simulink model "joint_trajectory_planner"  (R2020a)
settings: Solver=ode3  StartTime=0.0  StopTime=inf  FixedStep=0.01  RelTol=1e-3
libraries: robotlib x20, robotcorelib x1
settings Model: Creator=paolo  LastModifiedBy=paolo
settings OptimizationCC: EnhancedBackFolding=on  PassReuseOutputArgsAs=Individual arguments  ZeroExternalMemoryAtStartup=off  ZeroInternalMemoryAtStartup=off  MaxStackSize=64  OptimizeBlockOrder=speed  DifferentSizesBufferReuse=on  OptimizationCustomize=off  EfficientTunableParamExpr=on
settings DebuggingCC: ParameterTunabilityLossMsg=error
settings HardwareCC: ProdBitPerPointer=32  ProdBitPerSizeT=32  ProdBitPerPtrDiffT=32  ProdLargestAtomicFloat=None  ProdIntDivRoundTo=Undefined  ProdEndianess=Unspecified  ProdWordSize=32  ProdHWDeviceType=Generic->Unspecified (assume 32-bit Generic)
settings SFSimCC: MATLABDynamicMemAlloc=off
settings RTWCC: SystemTargetFile=ert.tlc  HardwareBoard=Robot Operating System (ROS)  TemplateMakefile=ert_default_tmf  Toolchain=Catkin  TargetLang=C++
settings CodeAppCC: ForceParamTrailComments=on  IgnoreCustomStorageClasses=off  OperatorAnnotations=on  SimulinkDataObjDesc=on  SFDataObjDesc=on  InsertBlockDesc=on

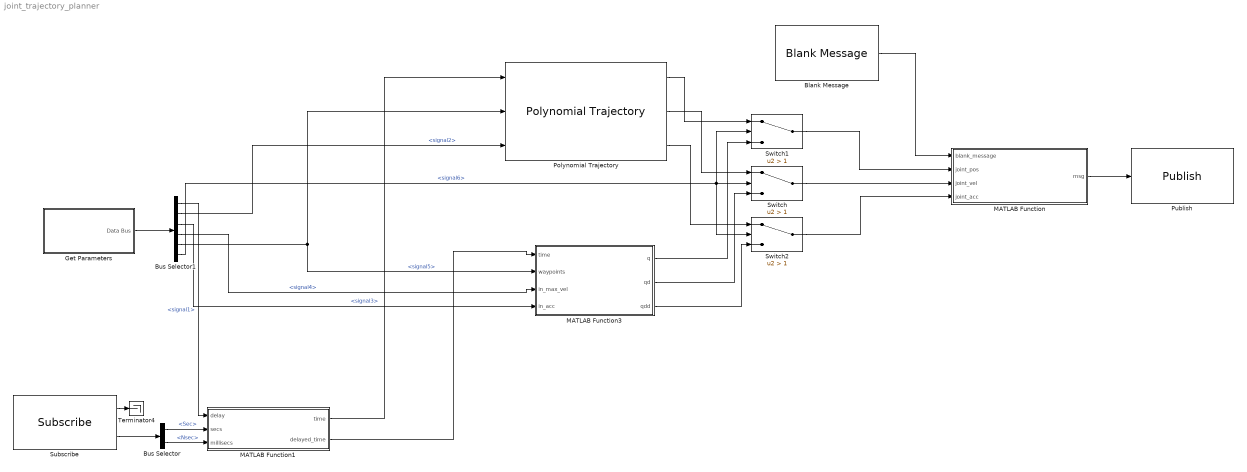
== system joint_trajectory_planner ==
  Blank Message : robotlib/Blank Message  messageClass=Message  entityType=trajectory_msgs/JointTrajectoryPoint  messageType=trajectory_msgs/JointTrajectoryPoint  SampleTime=-1
  Bus Selector : BusSelector  OutputSignals=Clock_.Sec,Clock_.Nsec
  Bus Selector1 : BusSelector  OutputSignals=signal1,signal2,signal3,signal4,signal5,signal6
  Get Parameters : Subsystem
  MATLAB Function : MATLAB Function  TreatAsAtomicUnit=on
  MATLAB Function1 : MATLAB Function  TreatAsAtomicUnit=on
  MATLAB Function3 : MATLAB Function  TreatAsAtomicUnit=on
  Polynomial Trajectory : robotcorelib/Polynomial Trajectory  WaypointSource=External  Waypoints=[ 0, 2, 1, 5, 0; -1, 3, 1, 4, 4 ]  TimePoints=[ 0, 1, 2, 3, 4 ]  TimeInterval=[ 1, 4 ]  Method=Cubic Polynomial  ParameterSource=Internal  VelocityBoundaryCondition=zeros( 6, 2 )  AccelerationBoundaryCondition=zeros( 2, 5 )  SimulateUsing=Interpreted execution
      settings: SourceProductBaseCode=NV,RO,RR
  Publish : robotlib/Publish  topicSource=Select from ROS network  topic=/joint_trajectory  messageType=trajectory_msgs/JointTrajectoryPoint  messageQueueLength=1
      link override SinkBlock: ROSTopic=/joint_trajectory  ROSMessageType=trajectory_msgs/JointTrajectoryPoint  SLBusName=SL_Bus_joint_trajectory_planner_JointTrajectoryPoint_y0wep  ModelName=joint_trajectory_planner  BlockId=Pub_joint_trajectory_planner_5
  Subscribe : robotlib/Subscribe  topicSource=Specify your own  topic=/clock  messageType=rosgraph_msgs/Clock  sampleTime=-1  messageQueueLength=1
  Switch : Switch  Criteria=u2 > Threshold  Threshold=1
  Switch1 : Switch  Criteria=u2 > Threshold  Threshold=1
  Switch2 : Switch  Criteria=u2 > Threshold  Threshold=1
  Terminator4 : Terminator
  wires:
  MATLAB Function/1(msg) -> Publish/1
  MATLAB Function3/2(qd) -> Switch/3
  Subscribe/1 -> Terminator4/1
  Subscribe/2 -> Bus Selector/1
  Bus Selector/1 -> MATLAB Function1/2(secs)  "<Sec>"
  Bus Selector/2 -> MATLAB Function1/3(millisecs)  "<Nsec>"
  MATLAB Function1/1(time) -> Polynomial Trajectory/1
  MATLAB Function3/1(q) -> Switch1/3
  MATLAB Function3/3(qdd) -> Switch2/3
  Get Parameters/1(Data Bus) -> Bus Selector1/1
  Bus Selector1/1 -> MATLAB Function1/1(delay)  "<signal1>"
  Bus Selector1/2 -> Polynomial Trajectory/3  "<signal2>"
  Bus Selector1/5 -> MATLAB Function3/2(waypoints), Polynomial Trajectory/2  "<signal5>"
  Blank Message/1 -> MATLAB Function/1(blank_message)
  Switch1/1 -> MATLAB Function/2(joint_pos)
  Switch/1 -> MATLAB Function/3(joint_vel)
  Switch2/1 -> MATLAB Function/4(joint_acc)
  Polynomial Trajectory/2 -> Switch/1
  Polynomial Trajectory/3 -> Switch2/1
  Bus Selector1/6 -> Switch2/2, Switch1/2, Switch/2  "<signal6>"
  MATLAB Function1/2(delayed_time) -> MATLAB Function3/1(time)
  Bus Selector1/4 -> MATLAB Function3/3(in_max_vel)  "<signal4>"
  Polynomial Trajectory/1 -> Switch1/1
  Bus Selector1/3 -> MATLAB Function3/4(in_acc)  "<signal3>"

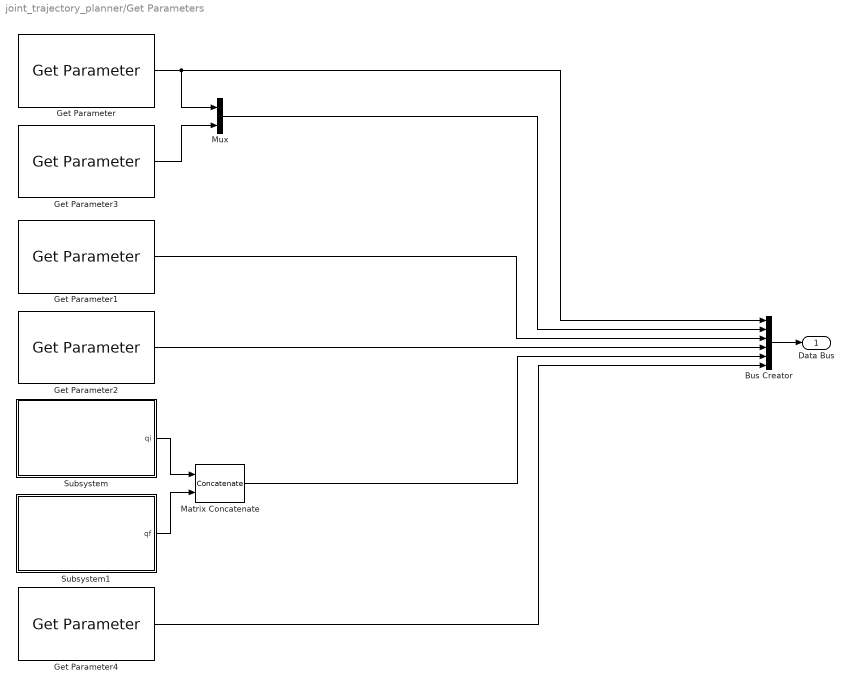
== system joint_trajectory_planner/Get Parameters ==
  Bus Creator : BusCreator  Inputs=6
  Get Parameter : robotlib/Get Parameter  ParameterSource=Specify your own  ParameterName=/start_delay  ParameterType=double  ParameterMaxArrayLength=16  ParameterInitialValue=20  SampleTime=-1  ShowErrorCodeOutput=off  ModelName=joint_trajectory_planner  BlockId=ParamGet_joint_trajectory_planner_26
      settings: SourceProductBaseCode=RR
  Get Parameter1 : robotlib/Get Parameter  ParameterSource=Specify your own  ParameterName=/max_ang_acc  ParameterType=double  ParameterMaxArrayLength=16  ParameterInitialValue=1  SampleTime=-1  ShowErrorCodeOutput=off  ModelName=joint_trajectory_planner  BlockId=ParamGet_joint_trajectory_planner_27
      settings: SourceProductBaseCode=RR
  Get Parameter2 : robotlib/Get Parameter  ParameterSource=Specify your own  ParameterName=/max_ang_vel  ParameterType=double  ParameterMaxArrayLength=16  ParameterInitialValue=1  SampleTime=-1  ShowErrorCodeOutput=off  ModelName=joint_trajectory_planner  BlockId=ParamGet_joint_trajectory_planner_28
      settings: SourceProductBaseCode=RR
  Get Parameter3 : robotlib/Get Parameter  ParameterSource=Specify your own  ParameterName=/tf  ParameterType=double  ParameterMaxArrayLength=16  ParameterInitialValue=60  SampleTime=-1  ShowErrorCodeOutput=off  ModelName=joint_trajectory_planner  BlockId=ParamGet_joint_trajectory_planner_49
      settings: SourceProductBaseCode=RR
  Get Parameter4 : robotlib/Get Parameter  ParameterSource=Specify your own  ParameterName=/trajectoryType  ParameterType=int32  ParameterMaxArrayLength=16  ParameterInitialValue=1  SampleTime=-1  ShowErrorCodeOutput=off  ModelName=joint_trajectory_planner  BlockId=ParamGet_joint_trajectory_planner_50
      settings: SourceProductBaseCode=RR
  Matrix Concatenate : Concatenate  Mode=Multidimensional array  ConcatenateDimension=2
  Mux : Mux  Inputs=2
  Subsystem : Subsystem
  Subsystem1 : Subsystem
  Data Bus : Outport
  wires:
  Subsystem/1(qi) -> Matrix Concatenate/1
  Subsystem1/1(qf) -> Matrix Concatenate/2
  Get Parameter/1 -> Bus Creator/1, Mux/1
  Get Parameter3/1 -> Mux/2
  Bus Creator/1 -> Data Bus/1
  Mux/1 -> Bus Creator/2
  Get Parameter1/1 -> Bus Creator/3
  Matrix Concatenate/1 -> Bus Creator/5
  Get Parameter4/1 -> Bus Creator/6
  Get Parameter2/1 -> Bus Creator/4

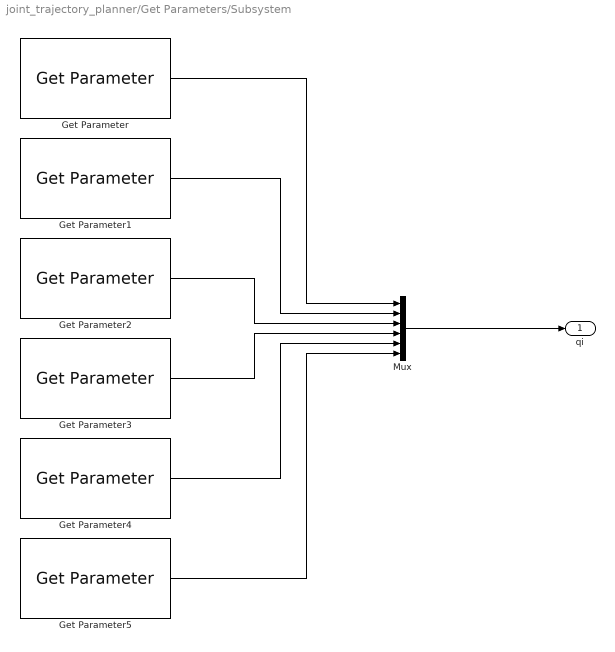
== system joint_trajectory_planner/Get Parameters/Subsystem ==
  Get Parameter : robotlib/Get Parameter  ParameterSource=Specify your own  ParameterName=/q1_initial  ParameterType=double  ParameterMaxArrayLength=16  ParameterInitialValue=0.0  SampleTime=-1  ShowErrorCodeOutput=off  ModelName=joint_trajectory_planner  BlockId=ParamGet_joint_trajectory_planner_34
      settings: SourceProductBaseCode=RR
  Get Parameter1 : robotlib/Get Parameter  ParameterSource=Specify your own  ParameterName=/q2_initial  ParameterType=double  ParameterMaxArrayLength=16  ParameterInitialValue=0.0  SampleTime=-1  ShowErrorCodeOutput=off  ModelName=joint_trajectory_planner  BlockId=ParamGet_joint_trajectory_planner_35
      settings: SourceProductBaseCode=RR
  Get Parameter2 : robotlib/Get Parameter  ParameterSource=Specify your own  ParameterName=/q3_initial  ParameterType=double  ParameterMaxArrayLength=16  ParameterInitialValue=0.0  SampleTime=-1  ShowErrorCodeOutput=off  ModelName=joint_trajectory_planner  BlockId=ParamGet_joint_trajectory_planner_36
      settings: SourceProductBaseCode=RR
  Get Parameter3 : robotlib/Get Parameter  ParameterSource=Specify your own  ParameterName=/q4_initial  ParameterType=double  ParameterMaxArrayLength=16  ParameterInitialValue=0.0  SampleTime=-1  ShowErrorCodeOutput=off  ModelName=joint_trajectory_planner  BlockId=ParamGet_joint_trajectory_planner_37
      settings: SourceProductBaseCode=RR
  Get Parameter4 : robotlib/Get Parameter  ParameterSource=Specify your own  ParameterName=/q5_initial  ParameterType=double  ParameterMaxArrayLength=16  ParameterInitialValue=0.0  SampleTime=-1  ShowErrorCodeOutput=off  ModelName=joint_trajectory_planner  BlockId=ParamGet_joint_trajectory_planner_38
      settings: SourceProductBaseCode=RR
  Get Parameter5 : robotlib/Get Parameter  ParameterSource=Specify your own  ParameterName=/q6_initial  ParameterType=double  ParameterMaxArrayLength=16  ParameterInitialValue=0.0  SampleTime=-1  ShowErrorCodeOutput=off  ModelName=joint_trajectory_planner  BlockId=ParamGet_joint_trajectory_planner_39
      settings: SourceProductBaseCode=RR
  Mux : Mux  Inputs=6
  qi : Outport
  wires:
  Get Parameter/1 -> Mux/1
  Get Parameter1/1 -> Mux/2
  Get Parameter2/1 -> Mux/3
  Get Parameter3/1 -> Mux/4
  Get Parameter4/1 -> Mux/5
  Get Parameter5/1 -> Mux/6
  Mux/1 -> qi/1

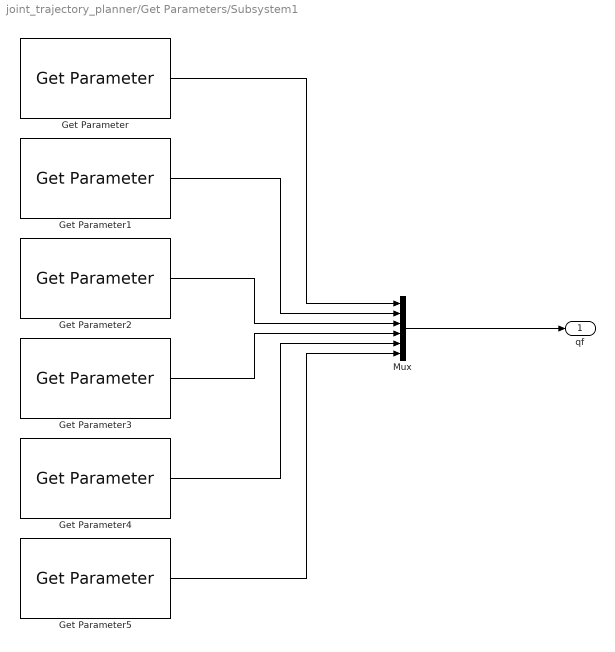
== system joint_trajectory_planner/Get Parameters/Subsystem1 ==
  Get Parameter : robotlib/Get Parameter  ParameterSource=Specify your own  ParameterName=/q1_final  ParameterType=double  ParameterMaxArrayLength=16  ParameterInitialValue=6.28  SampleTime=-1  ShowErrorCodeOutput=off  ModelName=joint_trajectory_planner  BlockId=ParamGet_joint_trajectory_planner_41
      settings: SourceProductBaseCode=RR
  Get Parameter1 : robotlib/Get Parameter  ParameterSource=Specify your own  ParameterName=/q2_final  ParameterType=double  ParameterMaxArrayLength=16  ParameterInitialValue=6.28  SampleTime=-1  ShowErrorCodeOutput=off  ModelName=joint_trajectory_planner  BlockId=ParamGet_joint_trajectory_planner_42
      settings: SourceProductBaseCode=RR
  Get Parameter2 : robotlib/Get Parameter  ParameterSource=Specify your own  ParameterName=/q3_final  ParameterType=double  ParameterMaxArrayLength=16  ParameterInitialValue=6.28  SampleTime=-1  ShowErrorCodeOutput=off  ModelName=joint_trajectory_planner  BlockId=ParamGet_joint_trajectory_planner_43
      settings: SourceProductBaseCode=RR
  Get Parameter3 : robotlib/Get Parameter  ParameterSource=Specify your own  ParameterName=/q4_final  ParameterType=double  ParameterMaxArrayLength=16  ParameterInitialValue=6.28  SampleTime=-1  ShowErrorCodeOutput=off  ModelName=joint_trajectory_planner  BlockId=ParamGet_joint_trajectory_planner_44
      settings: SourceProductBaseCode=RR
  Get Parameter4 : robotlib/Get Parameter  ParameterSource=Specify your own  ParameterName=/q5_final  ParameterType=double  ParameterMaxArrayLength=16  ParameterInitialValue=6.28  SampleTime=-1  ShowErrorCodeOutput=off  ModelName=joint_trajectory_planner  BlockId=ParamGet_joint_trajectory_planner_45
      settings: SourceProductBaseCode=RR
  Get Parameter5 : robotlib/Get Parameter  ParameterSource=Specify your own  ParameterName=/q6_final  ParameterType=double  ParameterMaxArrayLength=16  ParameterInitialValue=6.28  SampleTime=-1  ShowErrorCodeOutput=off  ModelName=joint_trajectory_planner  BlockId=ParamGet_joint_trajectory_planner_46
      settings: SourceProductBaseCode=RR
  Mux : Mux  Inputs=6
  qf : Outport
  wires:
  Get Parameter/1 -> Mux/1
  Get Parameter1/1 -> Mux/2
  Get Parameter2/1 -> Mux/3
  Get Parameter3/1 -> Mux/4
  Get Parameter4/1 -> Mux/5
  Get Parameter5/1 -> Mux/6
  Mux/1 -> qf/1

== matlab function joint_trajectory_planner/MATLAB Function1 ==
  data: delay input; secs input; time output; millisecs input; delayed_time output
function [time, delayed_time] = get_time(delay, secs, millisecs)

    time = secs + millisecs / 1e9;
    delayed_time = time - delay;
    
    if delayed_time < 0
        delayed_time = 0;
    end

== matlab function joint_trajectory_planner/MATLAB Function ==
  data: blank_message input; joint_pos input; msg output Bus: SL_Bus_joint_trajectory_planner_JointTrajectoryPoint_y0wep; joint_vel input; joint_acc input
function msg = assign_trajectory(blank_message, joint_pos, joint_vel, joint_acc)

    msg = blank_message;
    numJoints = length(joint_vel);
    msg.Velocities_SL_Info.CurrentLength = uint32(numJoints);
    msg.Velocities(1:numJoints) = joint_vel;
    msg.Positions_SL_Info.CurrentLength = uint32(numJoints);
    msg.Positions(1:numJoints) = joint_pos;
    msg.Accelerations_SL_Info.CurrentLength = uint32(numJoints);
    msg.Accelerations(1:numJoints) = joint_acc;

== matlab function joint_trajectory_planner/MATLAB Function3 ==
  data: time input; q output; waypoints input; in_max_vel input; in_acc input; qd output; qdd output
function [q, qd, qdd] = fcn(time, waypoints, in_max_vel, in_acc)

q_len = length(waypoints);

q = waypoints(:, 1);
qd = zeros(q_len, 1);
qdd = zeros(q_len, 1);

[rows, columns] = size(waypoints);

if length(in_max_vel) == 1
    max_vel = in_max_vel * ones(q_len, 1);
else
    max_vel = in_max_vel;
end

if length(in_acc) == 1
    acc = in_acc * ones(q_len, 1);
else
    acc = in_acc;
end

act_max_vel = zeros(rows, columns-1);
signes = zeros(rows, columns-1);
t = zeros(rows, columns-1, 3);

for i=1:rows
    
    t_up = max_vel(i) / acc(i);
   
    for j=1:columns-1
        
        dist = waypoints(i, j+1) - waypoints(i, j);
        signes(i, j) = sign(dist);
        
        if abs(dist) < t_up * max_vel(i)
            act_t_up = sqrt(abs(dist)/acc(i));
            t(i, j, 2) = 0;
            t(i, j, 1) = act_t_up;
            t(i, j, 3) = act_t_up;
            act_max_vel(i, j) = act_t_up * acc(i);
        else
            t(i, j, 1) = t_up;
            t(i, j, 3) = t_up;
            t(i, j, 2) = (abs(dist) - t_up * max_vel(i)) / max_vel(i);
            act_max_vel(i, j) = max_vel(i);
        end
        
    end
         
end

for i=1:rows
    
    t1 = time;
    
    for j=1:columns-1
        
        for k=1:3
            
            if t1 - t(i, j, k) < 0
                if k == 1
                    q(i) = q(i) + 1/2* acc(i) * t1^2 * signes(i, j);
                    qd(i) = acc(i) * t1 * signes(i, j);
                    qdd(i) = acc(i) * signes(i, j);
                    t1 = t1 - t(i, j, k);
                    break;
                end
                if k == 2
                    q(i) = q(i) + max_vel(i) * t1 * signes(i, j);
                    qd(i) = max_vel(i) * signes(i);
                    qdd(i) = 0;
                    t1 = t1 - t(i, j, k);
                    break;
                end
                q(i) = q(i) + (act_max_vel(j) * t1 - 1/2 * acc(i) * t1^2) * signes(i, j);
                qd(i) = (act_max_vel(i) - t1 * acc(i)) * signes(i, j);
                qdd(i) = - acc(i) * signes(i, j);
                t1 = t1 - t(i, j, k);
                break;
            end
            
            t1 = t1 - t(i, j, k);
            
            if k == 1
                q(i) = q(i) + 1/2 * acc(i) * t(i, j, k)^2 * signes(i, j);
                qd(i) = act_max_vel(i) * signes(i, j);
                qdd(i) = acc(i) * signes(i, j);
            elseif k == 2
                q(i) = q(i) + max_vel(i) * t(i, j, k) * signes(i, j);
                qd(i) = act_max_vel(i) * signes(i, j);
                qdd(i) = 0;
            else
                q(i) = q(i) + (act_max_vel(i) * t(i, j, k) - 1/2 * acc(i) * t(i, j, k)^2) * signes(i, j);
                qd(i) = 0;
                qdd(i) = 0;
            end
            
        if t1 < 0
            break   
        end
        
        end
        
    end
    
end

if time == 0
    qdd = zeros(q_len, 1);
end
